simulink model "COSTEP"  (R2024b)
settings: Solver=FixedStepAuto  StartTime=0.0  StopTime=25  FixedStep=1/3600  RelTol=1e-3
model workspace (MAT data in the model file):
  AD = Simulink.Parameter
  AD.Value = [1; 1; 1; 23.3; 33.9; 32.8; 49.9; 50.5]
  AD.Complexity = 'real'
  AD.Dimensions = [8 1]
  AD.DataType = 'auto'
  AG = Simulink.Parameter
  AG.Value = [3.411e-06; 3.799e-07; 2.491e-07; 3.567e-07; 3.463e-07; 3.93e-07; 1.7e-07; 1.5e-07]
  AG.Complexity = 'real'
  AG.Dimensions = [8 1]
  AG.Description = 'Coefficient A to determine Enthalpy
    | MBtu/lb·°F'
  AG.DataType = 'auto'
  AH = Simulink.Parameter
  AH.Value = [1e-06; 1e-06; 1e-06; 9.6e-07; 5.73e-07; 6.52e-07; 5.15e-07; 4.71e-07]
  AH.Complexity = 'real'
  AH.Dimensions = [8 1]
  AH.Description = 'Coefficient C to determine Enthalpy
    | MBtu/lb·°F³'
  AH.DataType = 'auto'
  AV = Simulink.Parameter
  AV.Value = [1e-06; 1e-06; 1e-06; 8.67e-05; 0.00016; 0.00016; 0.000225; 0.000209]
  AV.Complexity = 'real'
  AV.Dimensions = [8 1]
  AV.DataType = 'auto'
  AVP = Simulink.Parameter
  AVP.Value = [0; 0; 0; 15.92; 16.35; 16.35; 16.43; 17.21]
  AVP.Complexity = 'real'
  AVP.Dimensions = [8 1]
  AVP.DataType = 'auto'
  BCHL = Simulink.Parameter
  BCHL.Value = [0; 0; 0; 2118895; 2331760; 2492349; 2279927; 2994129]
  BCHL.Complexity = 'real'
  BCHL.Dimensions = [8 1]
  BCHL.DataType = 'auto'
  BCHV = Simulink.Parameter
  BCHV.Value = [254278; 948838; 625079; 1822034; 1979455; 2321416; 1491254; 1822996]
  BCHV.Complexity = 'real'
  BCHV.Dimensions = [8 1]
  BCHV.DataType = 'auto'
  BD = Simulink.Parameter
  BD.Value = [0; 0; 0; -0.07; -0.0957; -0.0995; -0.0191; -0.0541]
  BD.Complexity = 'real'
  BD.Dimensions = [8 1]
  BD.DataType = 'auto'
  BDIST = Simulink.Parameter
  BDIST.Value = 0
  BDIST.Complexity = 'real'
  BDIST.Dimensions = [1 1]
  BDIST.DataType = 'auto'
  BG = Simulink.Parameter
  BG.Value = [7.18e-10; 1.08e-09; 1.36e-11; 8.51e-10; 8.96e-10; 1.02e-09; 0; 0]
  BG.Complexity = 'real'
  BG.Dimensions = [8 1]
  BG.Description = 'Coefficient B to determine Enthalpy
    | MBtu/lb·°F²'
  BG.DataType = 'auto'
  BH = Simulink.Parameter
  BH.Value = [0; 0; 0; 8.7e-09; 2.41e-09; 2.18e-09; 5.65e-10; 8.7e-10]
  BH.Complexity = 'real'
  BH.Dimensions = [8 1]
  BH.Description = 'Coefficient B to determine Enthalpy
    | MBtu/lb·°F²'
  BH.DataType = 'auto'
  BVP = Simulink.Parameter
  BVP.Value = [0; 0; 0; -1444; -2114; -2114; -2748; -3318]
  BVP.Complexity = 'real'
  BVP.Dimensions = [8 1]
  BVP.DataType = 'auto'
  CD = Simulink.Parameter
  CD.Value = [0; 0; 0; -0.0002; -0.000152; -0.000233; -0.000425; -0.00015]
  CD.Complexity = 'real'
  CD.Dimensions = [8 1]
  CD.DataType = 'auto'
  CDIST = Simulink.Parameter
  CDIST.Value = 0
  CDIST.Complexity = 'real'
  CDIST.Dimensions = [1 1]
  CDIST.DataType = 'auto'
  CG = Simulink.Parameter
  CG.Value = [6e-13; -3.98e-13; -3.93e-14; -3.12e-13; -3.27e-13; -3.12e-13; 0; 0]
  CG.Complexity = 'real'
  CG.Dimensions = [8 1]
  CG.DataType = 'auto'
  CH = Simulink.Parameter
  CH.Value = [0; 0; 0; 4.81e-11; 1.82e-11; 1.94e-11; 3.82e-12; 2.62e-12]
  CH.Complexity = 'real'
  CH.Dimensions = [8 1]
  CH.DataType = 'auto'
  CVP = Simulink.Parameter
  CVP.Value = [0; 0; 0; 259; 265.5; 265.5; 232.9; 249.6]
  CVP.Complexity = 'real'
  CVP.Dimensions = [8 1]
  CVP.DataType = 'auto'
  DDIST = Simulink.Parameter
  DDIST.Value = 0
  DDIST.Complexity = 'real'
  DDIST.Dimensions = [1 1]
  DDIST.DataType = 'auto'
  DIST_CONST = Simulink.Parameter
  DIST_CONST.Value = [0.2  0.5  0.03  0.485  0; 0.7  1  0.003  0.005  0; 0.25  0.5  10  45  0; 0.7  1  10  45  0; 0.15  0.25  10  35  0; 0.15  0.25  10  40  0; 1  2  0.25  1  0; 1  2  0.25  1  0; 0.4  0.5  0.25  0  0; 1.5  2  0  0  0; 2  3  0  0  0; 1.5  2  0  0  0; 0.15  0.25  10  45  0; 0.25  0.5  10  45  0; 0.15  0.25  5  100  0; 0.25  0.5  20  400  0; 0.25  0.5  20  400  0; 0.7  1  75  1500  0; 0.1  0.2  50  1000  0; 0.1  0.2  60  1200  0]
  DIST_CONST.Complexity = 'real'
  DIST_CONST.Dimensions = [20 5]
  DIST_CONST.Description = 'The random variation disturbances make use of disturbance parameters that are 
    | used to define the characteristics of the disturbances over time. 
    | These disturbance parameters are defined here as a matrix where each row corresponds 
    | to a different disturbance number, and where each column represents the different 
    | disturbance parameters, i.e. HSPAN, HZERO, SSPAN, SZERO, SPSPAN'
  DIST_CONST.DataType = 'auto'
  ISV = Simulink.Parameter
  ISV.Value = [10.40491 4.364 7.57006 0.423 24.15513 2.9426 154.3771 159.1866 2.80852 63.75581 26.74026 46.38532 ... (350 elements, 50x7)]
  ISV.Complexity = 'real'
  ISV.Dimensions = [50 7]
  ISV.Description = 'Initial state variable value for the different mode selections'
  ISV.DataType = 'auto'
  TLAST = Simulink.Parameter
  TLAST.Value = 0
  TLAST.Complexity = 'real'
  TLAST.Dimensions = [1 1]
  TLAST.DataType = 'auto'
  TNEXT = Simulink.Parameter
  TNEXT.Value = 0.1
  TNEXT.Complexity = 'real'
  TNEXT.Dimensions = [1 1]
  TNEXT.DataType = 'auto'
  XMW = Simulink.Parameter
  XMW.Value = [2; 25.4; 28; 32; 46; 48; 62; 76]
  XMW.Complexity = 'real'
  XMW.Dimensions = [8 1]
  XMW.Description = 'Molecular Weight of components lb/lb-mol'
  XMW.DataType = 'auto'
  XNS = Simulink.Parameter
  XNS.Value = [0.0012; 18; 22; 0.05; 0.2; 0.21; 0.3; 0.5; 0.01; 0.0017; 0.01; 1; 0.3; 0.125; 1; 0.3; 0.115; 0.01; 1.15; 0.2; 0.01; 0.01; 0.25; 0.1; 0.25; 0.1; 0.25; 0.025; 0.25; 0.1; 0.25; 0.1; 0.25; 0.025; 0.05; 0.05; 0.01; 0.01; 0.01; 0.5; 0.5]
  XNS.Complexity = 'real'
  XNS.Dimensions = [41 1]
  XNS.DataType = 'auto'
  XNS2 = Simulink.Parameter
  XNS2.Value = [0.25; 0.1; 0.25; 0.1; 0.25; 0.025; 0.25; 0.1; 0.25; 0.1; 0.25; 0.025; 0.05; 0.05]
  XNS2.Complexity = 'real'
  XNS2.Dimensions = [14 1]
  XNS2.DataType = 'auto'
  XNS3 = Simulink.Parameter
  XNS3.Value = [0.01; 0.01; 0.01; 0.5; 0.5]
  XNS3.Complexity = 'real'
  XNS3.Dimensions = [5 1]
  XNS3.DataType = 'auto'
  XNSADD = Simulink.Parameter
  XNSADD.Value = [0.01; 0.01; 0.01; 0.01; 0.01; 0.125; 0.01; 0.125; 0.01; 0.01; 0.25; 0.1; 0.25; 0.1; 0.25; 0.025; 0.25; 0.1; 0.25; 0.1; 0.25; 0.025; 0.25; 0.1; 0.25; 0.1; 0.25; 0.025; 0.25; 0.1; 0.25; 0.1; 0.25; 0.025]
  XNSADD.Complexity = 'real'
  XNSADD.Dimensions = [34 1]
  XNSADD.DataType = 'auto'
  XNSE = Simulink.Parameter
  XNSE.Value = [0.01; 0.3; 0.01; 0.3; 0.01; 0.3; 0.01; 0.3; 0.01; 0.2; 0.01; 0.2; 0.3; 0.3; 0.01; 0.3; 0.2; 0.01; 0.3; 0.01; 0.3; 0.2; 0.01; 0.3]
  XNSE.Complexity = 'real'
  XNSE.Dimensions = [24 1]
  XNSE.DataType = 'auto'
undefined symbols (not defined in the file or in its folder): magnitude, msgbox, SETPT, XMEAS, XMV
libraries: mylib x381, dspindex x31
(part 1 of 12)
settings Model: Creator=j3vos  LastModifiedBy=bligr
settings SolverCC: AlgebraicLoopSolver=TrustRegion
settings DataIOCC: ReturnWorkspaceOutputs=off
settings DebuggingCC: UnconnectedInputMsg=warning  UnconnectedOutputMsg=warning  UnconnectedLineMsg=warning  ArithmeticOperatorsInVariantConditions=warning
settings ModelReferenceCC: EnableRefExpFcnMdlSchedulingChecks=on
settings SFSimCC: SimUseLocalCustomCode=off  CustomCodeUndefinedFunction=UseInterfaceOnly
settings RTWCC: RTWUseLocalCustomCode=off  GPUComputeCapability=3.5

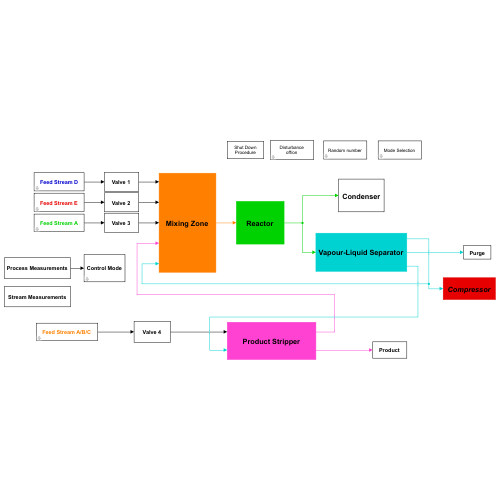
[thumbnail: Simulink's stored preview of the top-level diagram]
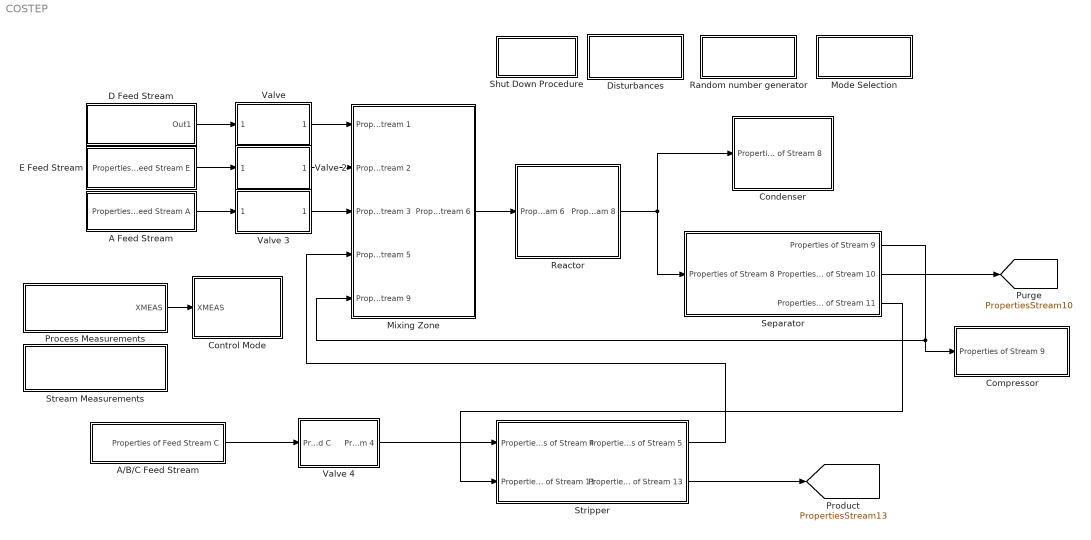
== system COSTEP ==
  A Feed Stream : Subsystem  mask{XST3_A=0.9999, XST3_B=0.0001, XST3_C=0, XST3_D=0, XST3_E=0, XST3_F=0, XST3_G=0, XST3_H=0, TST3=45, VRNG3=100}
      mask prompts: XST3_A "Fraction of A in Stream 3"; XST3_B "Fraction of B in Stream 3"; XST3_C "Fraction of C in Stream 3"; XST3_D "Fraction of D in Stream 3"; XST3_E "Fraction of E in Stream 3"; XST3_F "Fraction of F in Stream 3"; XST3_G "Fraction of G in Stream 3"; XST3_H "Fraction of H in Stream 3"; TST3 "Temperature of Stream 3"; VRNG3 "Maximum flow of Stream 3"
      mask DialogControl DescTextVar Prompt: Enter the Composition, Temperature and Mass Flow of Feed Stream A entering the plant
      mask DialogControl ParameterGroupVar Prompt: Properties of Feed Stream A
      mask Display: color('Green'),disp('{\bf\fontsize{12}Feed Stream A}', 'texmode','on');
  A/B/C Feed Stream : Subsystem  mask{XST4_A=0.485, XST4_B=0.005, XST4_C=0.51, XST4_D=0, XST4_E=0, XST4_F=0, XST4_G=0, XST4_H=0, TST4=45, VRNG4=1500}
      mask prompts: XST4_A "Fraction of A in Stream 4"; XST4_B "Fraction of B in Stream 4"; XST4_C "Fraction of C in Stream 4"; XST4_D "Fraction of D in Stream 4"; XST4_E "Fraction of E in Stream 4"; XST4_F "Fraction of F in Stream 4"; XST4_G "Fraction of G in Stream 4"; XST4_H "Fraction of H in Stream 4"; TST4 "Temperature of Stream 4"; VRNG4 "Maximum flow of Stream 4"
      mask DialogControl DescTextVar Prompt: Enter the Composition, Temperature and Mass Flow of Feed Stream C entering the plant
      mask DialogControl ParameterGroupVar Prompt: Properties of Feed Stream C
      mask Display: color('Orange'),disp('{\bf\fontsize{12}Feed Stream A/B/C}', 'texmode','on');
  Compressor : Subsystem
      mask Display: color('Black'),disp('{\bf\fontsize{16}Compressor}', 'texmode','on');
  Condenser : Subsystem
      mask Display: color('Black'),disp('{\bf\fontsize{16}Condenser}', 'texmode','on');
  Control Mode : Subsystem  mask{OPL=off, B=on, R=off, C=off, XMV1_0=63.053, XMV2_0=53.980, XMV3_0=24.644, XMV4_0=61.302, XMV5_0=22.210, XMV6_0=40.064, XMV7_0=38.100, XMV8_0=46.534, XMV9_0=47.446, XMV10_0=41.106, XMV11_0=18.114, XMV12_0=50.00000000}
      mask prompts: OPL "Open loop"; B "Braatz"; R "Ricker"; C "Custom"; XMV1_0 "Initial value of XMV(1) - D Feed flow valve"; XMV2_0 "Initial value of XMV(2) - E Feed flow valve"; XMV3_0 "Initial value of XMV(3) - A Feed flow valve"; XMV4_0 "Initial value of XMV(4) - A and C Feed flow valve"; XMV5_0 "Initial value of XMV(5) - Compressor recycle valve"; XMV6_0 "Initial value of XMV(6) - Purge valve"; XMV7_0 "Initial value of XMV(7) - Separator liquid flow valve"; XMV8_0 "Initial value of XMV(8) - Stripper liquid product flow valve"; XMV9_0 "Initial value of XMV(9) - Stripper steam valve"; XMV10_0 "Initial value of XMV(10) - Reactor cooling water flow valve"; XMV11_0 "Initial value of XMV(11) - Condenser cooling water flow valve"; XMV12_0 "Initial value of XMV(12) - Agitator speed"
      mask DialogControl DescGroupVar Prompt: Manipulated variables
      mask DialogControl DescTextVar Prompt: Control loops for manipulated variables. Open loop is the original TEP process without any control. Only one loop can be selected for a run. The base case values are the initial values of the manipulated variables
      mask DialogControl ParameterGroupVar Prompt: Control strategy
      mask DialogControl Container6 Prompt: Base case values
      mask Display: color('Black'),disp('{\bf\fontsize{12}Control Mode}', 'texmode','on');
  D Feed Stream : Subsystem  mask{XST1_A=0, XST1_B=0.0001, XST1_C=0, XST1_D=0.9999, XST1_E=0, XST1_F=0, XST1_G=0, XST1_H=0, TST1=45, VRNG1=400}
      mask prompts: XST1_A "Fraction of A in Stream 1"; XST1_B "Fraction of B in Stream 1"; XST1_C "Fraction of C in Stream 1"; XST1_D "Fraction of D in Stream 1"; XST1_E "Fraction of E in Stream 1"; XST1_F "Fraction of F in Stream 1"; XST1_G "Fraction of G in Stream 1"; XST1_H "Fraction of H in Stream 1"; TST1 "Temperature of Stream 1"; VRNG1 "Maximum flow of Stream 1"
      mask DialogControl DescTextVar Prompt: Enter the Composition, Temperature and Mass Flow of Feed Stream D entering the plant
      mask DialogControl ParameterGroupVar Prompt: Properties of Feed Stream D
      mask Display: color('Blue'),disp('{\bf\fontsize{12}Feed Stream D}', 'texmode','on');
  Disturbances : Subsystem  mask{DD=1, IDV1=off, IDV2=off, IDV3=off, IDV4=off, IDV5=off, IDV6=off, IDV7=off, IDV8=off, IDV9=off, IDV10=off, IDV11=off, IDV12=off, IDV13=off, IDV14=off, IDV15=off, IDV16=off, IDV17=off, IDV18=off, IDV19=off, IDV20=off, IDV21=off, IDV22=off, IDV23=off, IDV24=off, IDV25=off, IDV26=off, IDV27=off, IDV28=off}
      mask prompts: DD "Simulation time when disturbances should be introduced (in hours)"; IDV1 "IDV(1) - A/C feed ratio"; IDV2 "IDV(2) - B composition"; IDV3 "IDV(3) - D feed temperature"; IDV4 "IDV(4) - Reactor cooling water inlet temperature"; IDV5 "IDV(5) - Condenser cooling water inlet temperature"; IDV6 "IDV(6) - A feed loss"; IDV7 "IDV(7) - C header pressure loss (reduced availability)"; IDV8 "IDV(8) - A, B, C feed composition"; IDV9 "IDV(9) - D feed temperature"; IDV10 "IDV(10) - C feed temperature"; IDV11 "IDV(11) - Reactor cooling water inlet temperature"; IDV12 "IDV(12) - Condenser cooling water inlet temperature"; IDV13 "IDV(13) - Reaction kinetics"; IDV14 "IDV(14) - Reactor cooling water valve"; IDV15 "IDV(15) - Condenser cooling water valve"; IDV16 "IDV(16) - Unknown"; IDV17 "IDV(17) - Unknown"; IDV18 "IDV(18) - Unknown"; IDV19 "IDV(19) - Unknown"; IDV20 "IDV(20) - Unknown"; IDV21 "IDV(21) - A feed temperature"; IDV22 "IDV(22) - E feed temperature"; IDV23 "IDV(23) - A feed pressure"; IDV24 "IDV(24) - D feed pressure"; IDV25 "IDV(25) - E feed pressure"; IDV26 "IDV(26) - A, B, C feed pressure"; IDV27 "IDV(27) - Reactor cooling water supply pressure"; IDV28 "IDV(28) - Condensor cooling water supply pressure"
      mask DialogControl DescTextVar Prompt: Indicate if any disturbances are present (more than one can be ticked at a time)
      mask DialogControl ParameterGroupVar Prompt: Disturbances
      mask Display: color('Black'),disp('Disturbance\noff/on')
  E Feed Stream : Subsystem  mask{XST2_A=0, XST2_B=0, XST2_C=0, XST2_D=0, XST2_E=0.9999, XST2_F=0.0001, XST2_G=0, XST2_H=0, TST2=45, VRNG2=400}
      mask prompts: XST2_A "Fraction of A in Stream 2"; XST2_B "Fraction of B in Stream 2"; XST2_C "Fraction of C in Stream 2"; XST2_D "Fraction of D in Stream 2"; XST2_E "Fraction of E in Stream 2"; XST2_F "Fraction of F in Stream 2"; XST2_G "Fraction of G in Stream 2"; XST2_H "Fraction of H in Stream 2"; TST2 "Temperature of Stream 2"; VRNG2 "Maximum flow of Stream 2"
      mask DialogControl DescTextVar Prompt: Enter the Composition, Temperature and Mass Flow of Feed Stream E entering the plant
      mask DialogControl ParameterGroupVar Prompt: Properties of Feed Stream E
      mask Display: color('Red'),disp('{\bf\fontsize{12}Feed Stream E}', 'texmode','on');
  Mixing Zone : Subsystem
      mask Display: color('Black'),disp('{\bf\fontsize{16}Mixing Zone}', 'texmode','on');
  Mode Selection : Subsystem  mask{M=Mode - Original}
      mask prompts: M "Mode selection"
      mask DialogControl DescTextVar Prompt: Enter the mode for simulation run
      mask Display: disp('Mode Selection')
  Process Measurements : Subsystem
      mask Display: color('Black'),disp('{\bf\fontsize{12}Process Measurements}', 'texmode','on');
  Random number generator : Subsystem  mask{G=4243534565}
      mask prompts: G "Random number seed"
      mask DialogControl DescTextVar Prompt: Enter a random number so that every runs results will differ
      mask DialogControl ParameterGroupVar Prompt: Random Number Generator
      mask Display: disp('Random number')
  Reactor : Subsystem
      mask Display: color('Black'),disp('{\bf\fontsize{16}Reactor}', 'texmode','on');
  Separator : Subsystem
      mask Display: color('Black'),disp('{\bf\fontsize{16}Vapour-Liquid Separator}', 'texmode','on');
  Shut Down Procedure : Subsystem
      mask Display: color('black'),disp('Shut Down\nProcedure')
  Stream Measurements : Subsystem
      mask Display: color('Black'),disp('{\bf\fontsize{12}Stream Measurements}', 'texmode','on');
  Stripper : Subsystem
      mask Display: color('Black'),disp('{\bf\fontsize{16}Product Stripper}', 'texmode','on');
  Valve : Subsystem
      mask Display: color('Black'),disp('{\bf\fontsize{12}Valve 1}', 'texmode','on');
  Valve 2 : Subsystem
      mask Display: color('Black'),disp('{\bf\fontsize{12}Valve 2}', 'texmode','on');
  Valve 3 : Subsystem
      mask Display: color('Black'),disp('{\bf\fontsize{12}Valve 3}', 'texmode','on');
  Valve 4 : Subsystem
      mask Display: color('Black'),disp('{\bf\fontsize{12}Valve 4}', 'texmode','on');
  tag scope: PropertiesStream10=global, PropertiesStream13=global
  wires:
  Valve/1(Properties of Stream 1) -> Mixing Zone/1(Properties of Stream 1)
  E Feed Stream/1("Properties of Feed Stream E ") -> Valve 2/1(Properties of Feed E)
  Valve 2/1(Properties of Stream 2) -> Mixing Zone/2(Properties of Stream 2)
  A Feed Stream/1("Properties of Feed Stream A ") -> Valve 3/1(Properties of Feed A)
  Valve 3/1(Properties of Stream 3) -> Mixing Zone/3(Properties of Stream 3)
  Stripper/1(Properties of Stream 5) -> Mixing Zone/4(Properties of Stream 5)
  Mixing Zone/1(Properties of Stream 6) -> Reactor/1(Properties of Stream 6)
  A/B/C Feed Stream/1("Properties of Feed Stream C ") -> Valve 4/1(Properties of Feed C)
  Valve 4/1(Properties of Stream 4) -> Stripper/1(Properties of Stream 4)
  Separator/3(Properties of Stream 11) -> Stripper/2(Properties of Stream 11)
  Reactor/1(Properties of Stream 8) -> Separator/1(Properties of Stream 8), Condenser/1(Properties of Stream 8)
  Separator/1(Properties of Stream 9) -> Compressor/1(Properties of Stream 9), Mixing Zone/5(Properties of Stream 9)
  D Feed Stream/1(Out1) -> Valve/1(Properties of Feed D)
  Process Measurements/1(XMEAS) -> Control Mode/1(XMEAS)
  Stripper/2(Properties of Stream 13) -> [PropertiesStream13]
  Separator/2(Properties of Stream 10) -> [PropertiesStream10]

== system COSTEP/A Feed Stream ==
  Bus Creator : BusCreator  Inputs=4
  HST(3) Molar Enthalpy of Stream 3 MBtu/lb-mol : Subsystem
  TST(3) Temperature of Stream 3 °C : Subsystem
  VRNG(3) Max flow of Stream 3 through valve lb-mol/h : Subsystem
  XST(I,3) Composition of Stream 3 : Constant  Value=[XST3_A;XST3_B;XST3_C;XST3_D;XST3_E;XST3_F;XST3_G;XST3_H]
  "Properties of Feed Stream A " : Outport  VectorParamsAs1DForOutWhenUnconnected=off
  wires:
  XST(I,3) Composition of Stream 3/1 -> HST(3) Molar Enthalpy of Stream 3 MBtu/lb-mol/2(XST(I,3)), Bus Creator/1  "XST(I;3)"
  TST(3) Temperature of Stream 3 °C/1(TST(3)) -> HST(3) Molar Enthalpy of Stream 3 MBtu/lb-mol/1(TST(3)), Bus Creator/2  "TST(3)"
  VRNG(3) Max flow of Stream 3 through valve lb-mol/h/1(VRNG(3)) -> Bus Creator/3  "VRNG(3)"
  HST(3) Molar Enthalpy of Stream 3 MBtu/lb-mol/1(HST(3)) -> Bus Creator/4  "HST(3)"
  Bus Creator/1 -> "Properties of Feed Stream A "/1

== system COSTEP/A//B//C Feed Stream ==
  note: TST(4)
      | Temperature of Stream 4
      | °C
  Bus Creator : BusCreator  Inputs=4
  Bus Selector : BusSelector  OutputSignals=signal1.TESUB8(1),signal1.TESUB8(2)
  Bus Selector1 : BusSelector  OutputSignals=IDV(1),IDV(2)
  Bus Selector2 : BusSelector  OutputSignals=signal1.TESUB8(4)
  Gain : Gain
  HST(4) Molar Enthalpy of Stream 4 MBtu/lb-mol : Subsystem
  VRNG(4) Max flow of Stream 4 through valve lb-mol/h : Subsystem
  "XST(I;4) Composition of Stream 4 " : Subsystem
  "Properties of Feed Stream C " : Outport  VectorParamsAs1DForOutWhenUnconnected=off
  wires:
  "XST(I;4) Composition of Stream 4 "/1(XST(I;4)) -> HST(4) Molar Enthalpy of Stream 4 MBtu/lb-mol/2(XST(I,4)), Bus Creator/1  "XST(I;4)"
  Bus Selector2/1 -> Gain/1, HST(4) Molar Enthalpy of Stream 4 MBtu/lb-mol/1(TST(4))  "<TESUB8(4)>"
  VRNG(4) Max flow of Stream 4 through valve lb-mol/h/1(VRNG(4)) -> Bus Creator/3  "VRNG(4)"
  Bus Creator/1 -> "Properties of Feed Stream C "/1
  HST(4) Molar Enthalpy of Stream 4 MBtu/lb-mol/1(HST(4)) -> Bus Creator/4  "HST(4)"
  Bus Selector/2 -> "XST(I;4) Composition of Stream 4 "/2(TESUB8(2))  "<TESUB8(2)>"
  [TESUB8] -> Bus Selector2/1, Bus Selector/1
  Bus Selector/1 -> "XST(I;4) Composition of Stream 4 "/1(TESUB8(1))  "<TESUB8(1)>"
  [IDV] -> Bus Selector1/1
  Bus Selector1/1 -> "XST(I;4) Composition of Stream 4 "/3(IDV(1))  "<IDV(1)>"
  Bus Selector1/2 -> "XST(I;4) Composition of Stream 4 "/4(IDV(2))  "<IDV(2)>"
  Gain/1 -> Bus Creator/2  "TST(4)"

== system COSTEP/Compressor ==
  Properties of Stream 9 : Inport
  "  " : Subsystem
  Bus Selector : BusSelector  OutputSignals=XMWS(9)
  CPDH Compressor work MBtu/h : Subsystem
  CPFLMX : Constant  Value=280275
  Subsystem : Subsystem
  Subsystem1 : Subsystem
  TKS Temperature of Separator K : Sum
  To Convert °C to K : Constant  Value=273.15
  tag scope: CPDH=global, FLMS=global
  wires:
  Subsystem1/1(FLCOEF) -> "  "/3(FLCOEF)
  Subsystem/1(PR) -> "  "/1(PR)
  CPFLMX/1 -> "  "/2(CPFLMX), Subsystem1/1(CPFLMX)
  CPDH Compressor work MBtu/h/1(CPDH) -> [CPDH]
  "  "/1(FLMS) -> [FLMS], CPDH Compressor work MBtu/h/1(FLMS)
  TKS Temperature of Separator K/1 -> CPDH Compressor work MBtu/h/2(TKS)
  [TCS] -> TKS Temperature of Separator K/1
  To Convert °C to K/1 -> TKS Temperature of Separator K/2
  Properties of Stream 9/1 -> Bus Selector/1
  Bus Selector/1 -> CPDH Compressor work MBtu/h/3("XMWS(9) ")  "<XMWS(9)>"

== system COSTEP/Condenser ==
  Properties of Stream 8 : Inport
  Cooling water outlet temperature : Subsystem
  FWS Flow of cooling water to Condenser Gallons per minute : Subsystem
  Position of Valve 11 % : Subsystem
  Subsystem : Subsystem
  VRNG(11) Max flow of water through valve Gallons per minute : Subsystem
  tag scope: FWS=global, QUS=global
  wires:
  VRNG(11) Max flow of water through valve Gallons per minute/1(VRNG(11)) -> FWS Flow of cooling water to Condenser Gallons per minute/2(VRNG(11))
  FWS Flow of cooling water to Condenser Gallons per minute/1(FWS) -> [FWS], Cooling water outlet temperature/1(FWS)
  Position of Valve 11 %/1("YY(49) ") -> FWS Flow of cooling water to Condenser Gallons per minute/1(VPOS(11))
  Subsystem/1("QUS ") -> Cooling water outlet temperature/2(QUS), [QUS]
  Properties of Stream 8/1 -> Subsystem/1(Properties of Stream 8)
  Cooling water outlet temperature/1("YY(38) ") -> Subsystem/2(TWS)

== system COSTEP/Control Mode ==
  XMEAS : Inport
  Braatz : Subsystem
  Constant : Constant  Value=OPL
  Constant1 : Constant  Value=B
  Constant2 : Constant  Value=R
  Constant3 : Constant  Value=C
  Custom Controller : Subsystem
  Custom Controller1 : Subsystem
  If : If  NumInputs=4  IfExpression=u1 == 1  ElseIfExpressions=u2 == 1, u3 == 1, u4 == 1  ShowElse=off
  If Action Subsystem : Subsystem  TreatAsAtomicUnit=on
  If Action Subsystem1 : Subsystem  TreatAsAtomicUnit=on
  If Action Subsystem2 : Subsystem  TreatAsAtomicUnit=on
  If Action Subsystem3 : Subsystem  TreatAsAtomicUnit=on
  Merge : Merge  Inputs=4
  Open loop : Subsystem
  Subsystem : Subsystem
      mask Display: color('Black'),disp('Multi loop\nselection')
  To Workspace2 : ToWorkspace  VariableName=XMV  SampleTime=-1
  tag scope: XMV=global
  wires:
  Constant/1 -> Subsystem/1(OPL), If/1
  Constant1/1 -> Subsystem/2(B), If/2
  Constant2/1 -> Subsystem/3(R), If/3
  Merge/1 -> [XMV], To Workspace2/1
  If/1 -> If Action Subsystem/Action
  Open loop/1(XMV) -> If Action Subsystem/1(In1)
  If Action Subsystem1/1(Out1) -> Merge/2
  If/2 -> If Action Subsystem1/Action
  If/3 -> If Action Subsystem2/Action
  If Action Subsystem/1(Out1) -> Merge/1
  If Action Subsystem2/1(Out1) -> Merge/3
  Braatz/1(XMV) -> If Action Subsystem1/1(In1)
  Custom Controller1/1(XMV) -> If Action Subsystem2/1(In1)
  XMEAS/1 -> Braatz/1(XMEAS)
  If/4 -> If Action Subsystem3/Action
  Constant3/1 -> Subsystem/4(C), If/4
  Custom Controller/1(XMV) -> If Action Subsystem3/1(XMV)
  If Action Subsystem3/1(Out1) -> Merge/4

== system COSTEP/D Feed Stream ==
  Bus Creator : BusCreator  Inputs=4
  HST(1) Molar Enthalpy of Stream 1 MBtu/lb-mol : Subsystem
  TST(1) Temperature of Stream 1 °C : Subsystem
  VRNG(1) Max flow of Stream 1 through valve lb-mol/h : Subsystem
  XST(I,1) Composition of Stream 1 : Constant  Value=[XST1_A;XST1_B;XST1_C;XST1_D;XST1_E;XST1_F;XST1_G;XST1_H]
  Out1 : Outport  VectorParamsAs1DForOutWhenUnconnected=off
  wires:
  XST(I,1) Composition of Stream 1/1 -> HST(1) Molar Enthalpy of Stream 1 MBtu/lb-mol/2(XST(I,1)), Bus Creator/1  "XST(I;1)"
  VRNG(1) Max flow of Stream 1 through valve lb-mol/h/1(VRNG(1)) -> Bus Creator/3  "VRNG(1)"
  HST(1) Molar Enthalpy of Stream 1 MBtu/lb-mol/1(HST(1)) -> Bus Creator/4  "HST(1)"
  TST(1) Temperature of Stream 1 °C/1(TST(1)) -> Bus Creator/2, HST(1) Molar Enthalpy of Stream 1 MBtu/lb-mol/1(TST(1))
  Bus Creator/1 -> Out1/1

== system COSTEP/Disturbances ==
  Constant : Constant  Value=DD
  Delay : Delay  DelayLengthSource=Input port  DelayLength=1  DelayLengthUpperLimit=DD*3600  InitialCondition=0
      settings: InputPortMap=u0,p1
  Gain : Gain  Gain=3600
  IDV bus signal : Subsystem
  IDV from check box : Subsystem
  MATLAB Function : MATLAB Function  TreatAsAtomicUnit=on
  tag scope: IDV=global
  wires:
  Constant/1 -> Gain/1
  Gain/1 -> Delay/2
  Delay/1 -> [IDV]
  IDV from check box/1(Out1) -> MATLAB Function/1(IDV)
  MATLAB Function/1(IDV_out) -> IDV bus signal/1(IDV)
  IDV bus signal/1(Out1) -> Delay/1

== system COSTEP/E Feed Stream ==
  Bus Creator : BusCreator  Inputs=4
  HST(2) Molar Enthalpy of Stream 2 MBtu/lb-mol : Subsystem
  TST(2) Temperature of Stream 2 °C : Subsystem
  VRNG(2) Max flow of Stream 2 through valve lb-mol/h : Subsystem
  XST(I,2) Composition of Stream 2 : Constant  Value=[XST2_A;XST2_B;XST2_C;XST2_D;XST2_E;XST2_F;XST2_G;XST2_H]
  "Properties of Feed Stream E " : Outport  VectorParamsAs1DForOutWhenUnconnected=off
  wires:
  XST(I,2) Composition of Stream 2/1 -> HST(2) Molar Enthalpy of Stream 2 MBtu/lb-mol/2(XST(I,2)), Bus Creator/1  "XST(I;2)"
  TST(2) Temperature of Stream 2 °C/1(TST(2)) -> HST(2) Molar Enthalpy of Stream 2 MBtu/lb-mol/1(TST(2)), Bus Creator/2  "TST(2)"
  VRNG(2) Max flow of Stream 2 through valve lb-mol/h/1(VRNG(2)) -> Bus Creator/3  "VRNG(2)"
  Bus Creator/1 -> "Properties of Feed Stream E "/1
  HST(2) Molar Enthalpy of Stream 2 MBtu/lb-mol/1(HST(2)) -> Bus Creator/4  "HST(2)"

== system COSTEP/Mixing Zone ==
  Properties of Stream 1 : Inport
  Properties of Stream 2 : Inport  Port=2
  Properties of Stream 3 : Inport  Port=3
  Properties of Stream 5 : Inport  Port=4
  Properties of Stream 9 : Inport  Port=5
  Bus Creator : BusCreator  Inputs=2
  ETV Internal energy of Mixing zone Btu : Gain
  Holdup of Components in Mixing Zone : Subsystem
  Internal energy of mixing zone : Subsystem
  PTV Total pressure of Mixing zone mmHg : Subsystem
  Stream 6 : Subsystem
  "TCV Initial Temperature in Mixing zone °C " : Subsystem
  Properties of Stream 6 : Outport  VectorParamsAs1DForOutWhenUnconnected=off
  tag scope: PTV=global, PropertiesStream6=global
  wires:
  "TCV Initial Temperature in Mixing zone °C "/1(TCV) -> PTV Total pressure of Mixing zone mmHg/2(TCV), Stream 6/2(TST(6))
  Internal energy of mixing zone/1("YY(36) ") -> ETV Internal energy of Mixing zone Btu/1
  Properties of Stream 1/1 -> Holdup of Components in Mixing Zone/1(Properties of Stream 1), Internal energy of mixing zone/1(Properties of Stream 1)
  Properties of Stream 2/1 -> Internal energy of mixing zone/2(Properties of Stream 2), Holdup of Components in Mixing Zone/2(Properties of Stream 2)
  Properties of Stream 3/1 -> Internal energy of mixing zone/3(Properties of Stream 3), Holdup of Components in Mixing Zone/3(Properties of Stream 3)
  Stream 6/1(Properties of Stream 6) -> Bus Creator/1, Properties of Stream 6/1
  Properties of Stream 5/1 -> Internal energy of mixing zone/4(Properties of Stream 5), Holdup of Components in Mixing Zone/4(Properties of Stream 5)
  Properties of Stream 9/1 -> Internal energy of mixing zone/5(Properties of Stream 9), Holdup of Components in Mixing Zone/5(Properties of Stream 9)
  Holdup of Components in Mixing Zone/1(XVV) -> Stream 6/1(XST(I,6)), "TCV Initial Temperature in Mixing zone °C "/3(XVV)
  Holdup of Components in Mixing Zone/2(UTVV) -> PTV Total pressure of Mixing zone mmHg/1(UTVV), "TCV Initial Temperature in Mixing zone °C "/1(UTVV)
  PTV Total pressure of Mixing zone mmHg/1(PTV) -> Bus Creator/2, [PTV]  "PTV"
  Bus Creator/1 -> [PropertiesStream6]
  ETV Internal energy of Mixing zone Btu/1 -> "TCV Initial Temperature in Mixing zone °C "/2(ETV)

== system COSTEP/Mode Selection ==
  Constant : Constant  Value=M
  MATLAB Function : MATLAB Function  TreatAsAtomicUnit=on
  tag scope: M=global
  wires:
  Constant/1 -> MATLAB Function/1(M)
  MATLAB Function/1(M_out) -> [M]

== system COSTEP/Process Measurements ==
  Bus Creator1 : BusCreator  Inputs=10
  Compressor Work : Subsystem
  Condenser Cooling Outlet Water Temperature : Subsystem
  Feed Streams : Subsystem
  Product analysis : Subsystem
  Purge gas analysis : Subsystem
  Reactor Cooling Outlet Water Temperature : Subsystem
  Reactor feed analysis : Subsystem
  Subsystem3 : Subsystem
  Subsystem4 : Subsystem
  Subsystem5 : Subsystem
  To Workspace1 : ToWorkspace  VariableName=XMEAS  SampleTime=-1
  XMEAS : Outport  VectorParamsAs1DForOutWhenUnconnected=off
  tag scope: XMEAS=global
  wires:
  Bus Creator1/1 -> To Workspace1/1, [XMEAS], XMEAS/1
  Feed Streams/1(XMEASF) -> Bus Creator1/1
  Subsystem3/1(Reactor) -> Bus Creator1/2
  Subsystem4/1(Separator) -> Bus Creator1/3
  Subsystem5/1(Stripper) -> Bus Creator1/4
  Product analysis/1(XMEAS) -> Bus Creator1/10
  Purge gas analysis/1(XMEASP) -> Bus Creator1/9
  Reactor feed analysis/1(XMEASR) -> Bus Creator1/8
  Compressor Work/1("XMEAS(20) ") -> Bus Creator1/5
  Reactor Cooling Outlet Water Temperature/1(XMEAS(21)) -> Bus Creator1/6
  Condenser Cooling Outlet Water Temperature/1(XMEAS(22)) -> Bus Creator1/7

== system COSTEP/Random number generator ==
  Additional Stream Measurements : Delay  DelayLength=1  InitialConditionSource=Input port  InitialCondition=0
      settings: InputPortMap=u0,p4
  Bus Creator : BusCreator  Inputs=3
  Constant : Constant  Value=G
  "Disturbances 17, 18, 20 IDVWLK=10-12" : Subsystem
  "Disturbances 21, 22, 23, 24, 25, 26, 27, 28 IDVWLK=13-20" : Subsystem
  "Disturbances 8, 9, 10, 11, 12, 13, 16 IDVWLK=1-9" : Subsystem
  MATLAB Function : MATLAB Function  TreatAsAtomicUnit=on
  Original G : Delay  DelayLength=1  InitialConditionSource=Input port  InitialCondition=0
      settings: InputPortMap=u0,p4
  Process Disturbances : Delay  DelayLength=1  InitialConditionSource=Input port  InitialCondition=0
      settings: InputPortMap=u0,p4
  Process Measurements XMEAS(I) I=1-22 : Subsystem
  Process Measurements XMEAS(I) I=23-36 : Subsystem
  Process Measurements XMEAS(I) I=37-41 : Subsystem
  Stream Measurements SMEAS Gas analysis1 : Subsystem
  Stream Measurements SMEAS Product analysis1 : Subsystem
  Stream Measurements SMEAS1 : Subsystem
  tag scope: TESUB8=global
  wires:
  "Disturbances 17, 18, 20 IDVWLK=10-12"/1(G2) -> Process Measurements XMEAS(I) I=1-22/1(G2)
  Process Measurements XMEAS(I) I=37-41/1(G5) -> Original G/1
  Process Measurements XMEAS(I) I=1-22/1(G3) -> Process Measurements XMEAS(I) I=23-36/1(G3)
  Process Measurements XMEAS(I) I=23-36/1(G4) -> Process Measurements XMEAS(I) I=37-41/1(G4)
  "Disturbances 8, 9, 10, 11, 12, 13, 16 IDVWLK=1-9"/1(G1) -> "Disturbances 17, 18, 20 IDVWLK=10-12"/1(G1)
  Original G/1 -> "Disturbances 8, 9, 10, 11, 12, 13, 16 IDVWLK=1-9"/1(G)
  Bus Creator/1 -> [TESUB8]
  "Disturbances 8, 9, 10, 11, 12, 13, 16 IDVWLK=1-9"/2(Out1) -> Bus Creator/1
  "Disturbances 17, 18, 20 IDVWLK=10-12"/2(Out1) -> Bus Creator/2
  "Disturbances 21, 22, 23, 24, 25, 26, 27, 28 IDVWLK=13-20"/1(G1) -> Process Disturbances/1
  Process Disturbances/1 -> "Disturbances 21, 22, 23, 24, 25, 26, 27, 28 IDVWLK=13-20"/1(G)
  Constant/1 -> MATLAB Function/1(G)
  Stream Measurements SMEAS Product analysis1/1(GE4) -> Additional Stream Measurements/1
  Stream Measurements SMEAS1/1(G2E) -> Stream Measurements SMEAS Gas analysis1/1(GE2)
  Stream Measurements SMEAS Gas analysis1/1(GE3) -> Stream Measurements SMEAS Product analysis1/1(GE3)
  Additional Stream Measurements/1 -> Stream Measurements SMEAS1/1(G1E)
  MATLAB Function/1(G_out) -> Additional Stream Measurements/2, Process Disturbances/2, Original G/2
  "Disturbances 21, 22, 23, 24, 25, 26, 27, 28 IDVWLK=13-20"/2(Out1) -> Bus Creator/3

== system COSTEP/Reactor ==
  Properties of Stream 6 : Inport
  Bus Creator : BusCreator  Inputs=2
  Holdup of Components in Reactor : Subsystem
  Internal energy of reactor : Subsystem
  Pressure of Reactor : Subsystem
  Reaction Rates : Subsystem
  Reactor Heat exchanger : Subsystem
  Stream 8 : Subsystem
  "TCR Initial Temperature in Reactor °C " : Subsystem
  Total Vapour Component Holdup in Reactor : Subsystem
  Vapour Component Fraction in Reactor : Subsystem
  Volume of Reactor : Subsystem
  Properties of Stream 8 : Outport  VectorParamsAs1DForOutWhenUnconnected=off
  tag scope: PTR=global, PropertiesStream8=global, TCR=global, VLR=global
  wires:
  Holdup of Components in Reactor/1(UTLR) -> Volume of Reactor/2(UTLR), "TCR Initial Temperature in Reactor °C "/1(UTLR)
  Internal energy of reactor/1("YY(9) ") -> "TCR Initial Temperature in Reactor °C "/2(ETR)  "ETR Internal energy of reactor MBtu"
  Stream 8/1(Properties of Stream 8) -> Bus Creator/1, Properties of Stream 8/1
  Reactor Heat exchanger/1(QUR) -> Internal energy of reactor/2(QUR)
  Properties of Stream 6/1 -> Holdup of Components in Reactor/2(Properties of Stream 6), Internal energy of reactor/3(Properties of Stream 6)
  Reaction Rates/1("RH ") -> Internal energy of reactor/1(RH)
  Reaction Rates/2(CRXR) -> Holdup of Components in Reactor/1(CRXR)
  Holdup of Components in Reactor/2(XLR) -> Pressure of Reactor/1(XLR), "TCR Initial Temperature in Reactor °C "/3(XLR), Volume of Reactor/1(XLR)
  Holdup of Components in Reactor/3(UCVR) -> Pressure of Reactor/3(UCVR)
  Pressure of Reactor/2(PPR) -> Reaction Rates/2(PPR), Vapour Component Fraction in Reactor/1(PPR)
  Pressure of Reactor/1(PTR) -> Bus Creator/2, [PTR]  "PTR"
  "TCR Initial Temperature in Reactor °C "/1(TCR) -> Stream 8/1(TST(8)), [TCR]
  Volume of Reactor/1(VVR) -> Reaction Rates/1(VVR), Total Vapour Component Holdup in Reactor/1(VVR), Pressure of Reactor/2(VVR)
  Vapour Component Fraction in Reactor/1(XVR) -> Total Vapour Component Holdup in Reactor/2(XVR), Stream 8/2(XTS(I,8))
  Volume of Reactor/2(VLR) -> [VLR]
  Bus Creator/1 -> [PropertiesStream8]

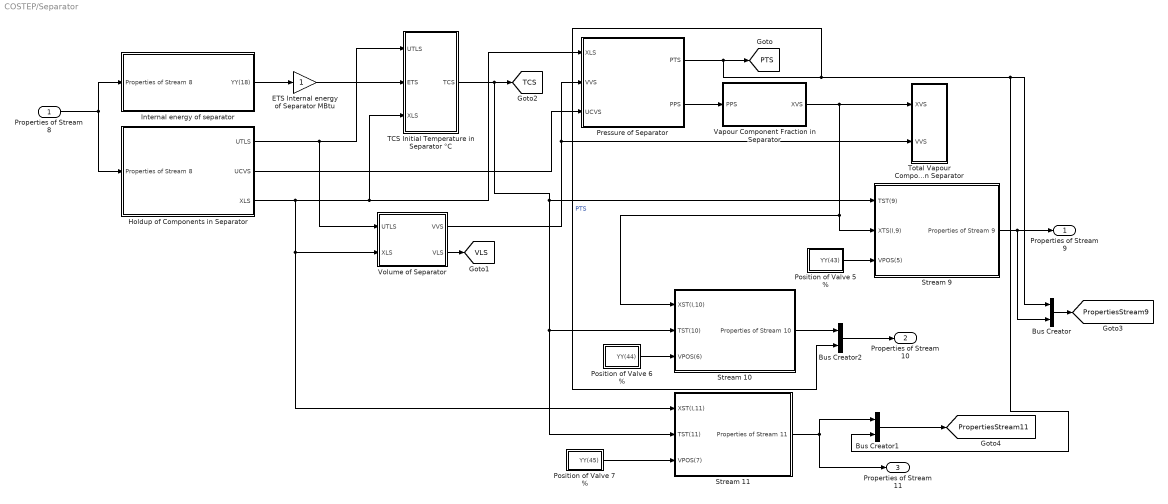
== system COSTEP/Separator ==
  Properties of Stream 8 : Inport
  Bus Creator : BusCreator  Inputs=2
  Bus Creator1 : BusCreator  Inputs=2
  Bus Creator2 : BusCreator  Inputs=2
  ETS Internal energy of Separator MBtu : Gain
  Holdup of Components in Separator : Subsystem
  Internal energy of separator : Subsystem
  Position of Valve 5 % : Subsystem
  Position of Valve 6 % : Subsystem
  Position of Valve 7 % : Subsystem
  Pressure of Separator : Subsystem
  Stream 10 : Subsystem
  Stream 11 : Subsystem
  Stream 9 : Subsystem
  "TCS Initial Temperature in Separator °C " : Subsystem
  Total Vapour Component Holdup in Separator : Subsystem
  Vapour Component Fraction in Separator : Subsystem
  Volume of Separator : Subsystem
  Properties of Stream 9 : Outport  VectorParamsAs1DForOutWhenUnconnected=off
  Properties of Stream 10 : Outport  Port=2  VectorParamsAs1DForOutWhenUnconnected=off
  Properties of Stream 11 : Outport  Port=3  VectorParamsAs1DForOutWhenUnconnected=off
  tag scope: PTS=global, PropertiesStream11=global, PropertiesStream9=global, TCS=global, VLS=global
  wires:
  Internal energy of separator/1("YY(18) ") -> ETS Internal energy of Separator MBtu/1
  Stream 9/1(Properties of Stream 9) -> Bus Creator/2, Properties of Stream 9/1
  Stream 11/1(Properties of Stream 11) -> Bus Creator1/1, Properties of Stream 11/1
  Holdup of Components in Separator/1(UTLS) -> Volume of Separator/1(UTLS), "TCS Initial Temperature in Separator °C "/1(UTLS)
  Holdup of Components in Separator/3(XLS) -> "TCS Initial Temperature in Separator °C "/3(XLS), Pressure of Separator/1(XLS), Stream 11/1(XST(I,11)), Volume of Separator/2(XLS)
  Volume of Separator/1(VVS) -> Pressure of Separator/2(VVS), Total Vapour Component Holdup in Separator/2(VVS)
  Volume of Separator/2(VLS) -> [VLS]
  Pressure of Separator/1(PTS) -> Bus Creator2/2, Bus Creator1/2, Bus Creator/1, [PTS]  "PTS"
  Holdup of Components in Separator/2(UCVS) -> Pressure of Separator/3(UCVS)
  Vapour Component Fraction in Separator/1(XVS) -> Stream 10/1(XST(I,10)), Stream 9/2(XTS(I,9)), Total Vapour Component Holdup in Separator/1(XVS)
  Pressure of Separator/2(PPS) -> Vapour Component Fraction in Separator/1(PPS)
  Properties of Stream 8/1 -> Internal energy of separator/1(Properties of Stream 8), Holdup of Components in Separator/1(Properties of Stream 8)
  Position of Valve 5 %/1("YY(43) ") -> Stream 9/3(VPOS(5))
  Position of Valve 6 %/1("YY(44) ") -> Stream 10/3(VPOS(6))
  Position of Valve 7 %/1("YY(45) ") -> Stream 11/3(VPOS(7))
  ETS Internal energy of Separator MBtu/1 -> "TCS Initial Temperature in Separator °C "/2(ETS)
  "TCS Initial Temperature in Separator °C "/1(TCS) -> [TCS], Stream 11/2(TST(11)), Stream 10/2(TST(10)), Stream 9/1(TST(9))
  Bus Creator/1 -> [PropertiesStream9]
  Bus Creator1/1 -> [PropertiesStream11]
  Stream 10/1(Properties of Stream 10) -> Bus Creator2/1
  Bus Creator2/1 -> Properties of Stream 10/1

== system COSTEP/Shut Down Procedure ==
  Add : Sum  Inputs=8  OutDataTypeStr=double  AccumDataTypeStr=double
  Reactor Level to High : Subsystem
  Reactor Level to Low : Subsystem
  Reactor Presssure to High : Subsystem
  Reactor Temperature to High : Subsystem
  Separator Level to High : Subsystem
  Separator Level to Low : Subsystem
  Stripper Level to High : Subsystem
  Stripper Level to Low : Subsystem
  tag scope: ISD=global
  wires:
  [VLR] -> Reactor Level to Low/1(VLR), Reactor Level to High/1(VLR)
  [VLS] -> Separator Level to Low/1(VLS), Separator Level to High/1(VLS)
  [VLC] -> Stripper Level to Low/1(VLC), Stripper Level to High/1(VLC)
  Reactor Presssure to High/1(ISD) -> Add/1
  Reactor Temperature to High/1(ISD) -> Add/2
  Reactor Level to High/1(ISD) -> Add/3
  Reactor Level to Low/1(ISD) -> Add/4
  Separator Level to High/1(ISD) -> Add/5
  Separator Level to Low/1(ISD) -> Add/6
  Stripper Level to High/1(ISD) -> Add/7
  Stripper Level to Low/1(ISD) -> Add/8
  Add/1 -> [ISD]

== system COSTEP/Stream Measurements ==
  Stream Variables : ToWorkspace  VariableName=SM  SampleTime=-1
  Subsystem6 : Subsystem
      mask Display: image('$imagefile'); % Use "Edit Image" on toolstrip to change.
  wires:
  Subsystem6/1(SM) -> Stream Variables/1

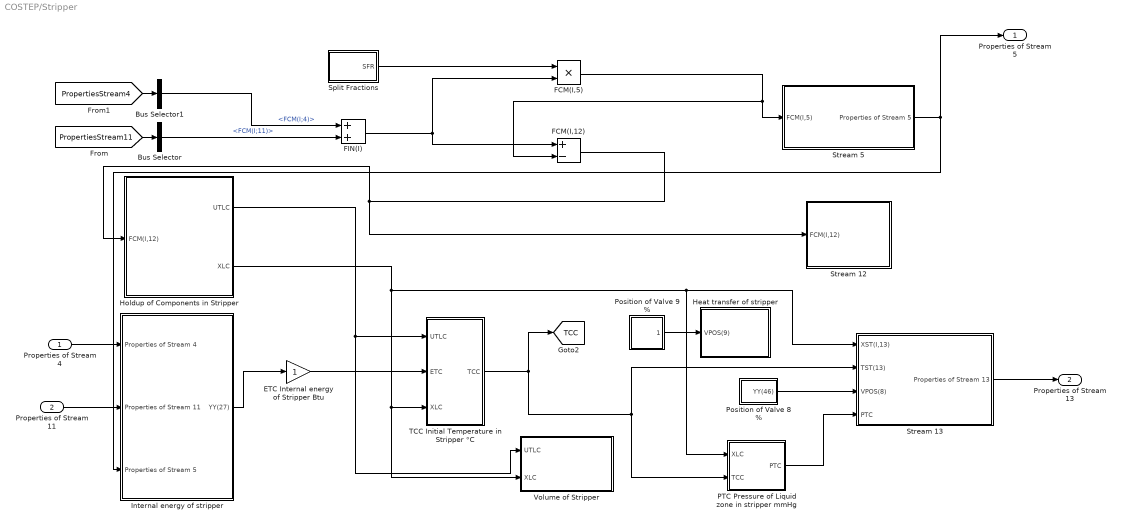
== system COSTEP/Stripper ==
  Properties of Stream 4 : Inport
  Properties of Stream 11 : Inport  Port=2
  Bus Selector : BusSelector  OutputSignals=signal1.FCM(I;11)
  Bus Selector1 : BusSelector  OutputSignals=FCM(I;4)
  ETC Internal energy of Stripper Btu : Gain
  FCM(I,12) : Sum  Inputs=+-
  FCM(I,5) : Product
  FIN(I) : Sum
  Heat transfer of stripper : Subsystem
  Holdup of Components in Stripper : Subsystem
  Internal energy of stripper : Subsystem
  PTC Pressure of Liquid zone in stripper mmHg : Subsystem
  Position of Valve 8 % : Subsystem
  Position of Valve 9 % : Subsystem
  Split Fractions : Subsystem
  Stream 12 : Subsystem
  Stream 13 : Subsystem
  Stream 5 : Subsystem
  "TCC Initial Temperature in Stripper °C " : Subsystem
  Volume of Stripper : Subsystem
  Properties of Stream 5 : Outport  VectorParamsAs1DForOutWhenUnconnected=off
  Properties of Stream 13 : Outport  Port=2  VectorParamsAs1DForOutWhenUnconnected=off
  tag scope: TCC=global
  wires:
  Holdup of Components in Stripper/1(UTLC) -> Volume of Stripper/1(UTLC), "TCC Initial Temperature in Stripper °C "/1(UTLC)
  Internal energy of stripper/1("YY(27) ") -> ETC Internal energy of Stripper Btu/1
  ETC Internal energy of Stripper Btu/1 -> "TCC Initial Temperature in Stripper °C "/2(ETC)
  "TCC Initial Temperature in Stripper °C "/1(TCC) -> [TCC], Stream 13/2(TST(13)), PTC Pressure of Liquid zone in stripper mmHg/2(TCC)
  FIN(I)/1 -> FCM(I,12)/1, FCM(I,5)/2
  FCM(I,5)/1 -> FCM(I,12)/2, Stream 5/1(FCM(I,5))
  FCM(I,12)/1 -> Holdup of Components in Stripper/1("FCM(I,12) "), Stream 12/1(FCM(I,12))
  Stream 13/1(Properties of Stream 13) -> Properties of Stream 13/1
  Stream 5/1(Properties of Stream 5) -> Properties of Stream 5/1, Internal energy of stripper/3(Properties of Stream 5)
  Properties of Stream 4/1 -> Internal energy of stripper/1(Properties of Stream 4)
  Properties of Stream 11/1 -> Internal energy of stripper/2(Properties of Stream 11)
  Position of Valve 9 %/1("YY(47) ") -> Heat transfer of stripper/1(VPOS(9))
  Split Fractions/1(SFR) -> FCM(I,5)/1
  [PropertiesStream11] -> Bus Selector/1
  Bus Selector/1 -> FIN(I)/2  "<FCM(I;11)>"
  [PropertiesStream4] -> Bus Selector1/1
  Bus Selector1/1 -> FIN(I)/1  "<FCM(I;4)>"
  Position of Valve 8 %/1("YY(46) ") -> Stream 13/3(VPOS(8))
  Holdup of Components in Stripper/2(XLC) -> "TCC Initial Temperature in Stripper °C "/3(XLC), Volume of Stripper/2(XLC), PTC Pressure of Liquid zone in stripper mmHg/1(XLC), Stream 13/1(XST(I,13))
  PTC Pressure of Liquid zone in stripper mmHg/1(PTC) -> Stream 13/4(PTC)

== system COSTEP/Valve ==
  Properties of Feed D : Inport
  Bus Creator : BusCreator  Inputs=5
  Bus Selector : BusSelector  OutputSignals=VRNG(1)
  Bus Selector1 : BusSelector  OutputSignals=XST(I;1),TST(1),HST(1)
  FCM(I,1) Component molar flow of Stream 1 lb-mol/h : Product  OutDataTypeStr=Inherit: Same as first input
  FTM(1) Total molar flow of Stream 1 lb-mol/h : Subsystem
  Position of Valve 1 % : Subsystem
  Properties of Stream 1 : Outport  VectorParamsAs1DForOutWhenUnconnected=off
  tag scope: PropertiesStream1=global
  wires:
  Position of Valve 1 %/1("YY(39) ") -> FTM(1) Total molar flow of Stream 1 lb-mol/h/1(VPOS(1))
  Properties of Feed D/1 -> Bus Selector1/1, Bus Selector/1
  Bus Selector/1 -> FTM(1) Total molar flow of Stream 1 lb-mol/h/2(VRNG(1))  "<VRNG(1)>"
  Bus Selector1/1 -> Bus Creator/1, FCM(I,1) Component molar flow of Stream 1 lb-mol/h/1  "<XST(I;1)>"
  FTM(1) Total molar flow of Stream 1 lb-mol/h/1(FTM(1)) -> Bus Creator/4, FCM(I,1) Component molar flow of Stream 1 lb-mol/h/2  "FTM(1)"
  Bus Selector1/2 -> Bus Creator/2  "<TST(1)>"
  Bus Selector1/3 -> Bus Creator/3  "<HST(1)>"
  FCM(I,1) Component molar flow of Stream 1 lb-mol/h/1 -> Bus Creator/5  "FCM(I;1)"
  Bus Creator/1 -> [PropertiesStream1], Properties of Stream 1/1

== system COSTEP/Valve 2 ==
  Properties of Feed E : Inport
  Bus Creator : BusCreator  Inputs=5
  Bus Selector : BusSelector  OutputSignals=VRNG(2)
  Bus Selector1 : BusSelector  OutputSignals=XST(I;2),TST(2),HST(2)
  FCM(I,2) Component molar flow of Stream 2 lb-mol/h : Product
  FTM(2) Total molar flow of Stream 2 lb-mol/h : Subsystem
  Position of Valve 2 % : Subsystem
  Properties of Stream 2 : Outport  VectorParamsAs1DForOutWhenUnconnected=off
  tag scope: PropertiesStream2=global
  wires:
  Properties of Feed E/1 -> Bus Selector1/1, Bus Selector/1
  Bus Selector/1 -> FTM(2) Total molar flow of Stream 2 lb-mol/h/2(VRNG(2))  "<VRNG(2)>"
  Bus Selector1/1 -> Bus Creator/1, FCM(I,2) Component molar flow of Stream 2 lb-mol/h/1  "<XST(I;2)>"
  FTM(2) Total molar flow of Stream 2 lb-mol/h/1(FTM(2)) -> Bus Creator/4, FCM(I,2) Component molar flow of Stream 2 lb-mol/h/2  "FTM(2)"
  Bus Selector1/2 -> Bus Creator/2  "<TST(2)>"
  Bus Selector1/3 -> Bus Creator/3  "<HST(2)>"
  FCM(I,2) Component molar flow of Stream 2 lb-mol/h/1 -> Bus Creator/5  "FCM(I;2)"
  Bus Creator/1 -> [PropertiesStream2], Properties of Stream 2/1
  Position of Valve 2 %/1("YY(40)  ") -> FTM(2) Total molar flow of Stream 2 lb-mol/h/1(VPOS(2))

== system COSTEP/Valve 3 ==
  Properties of Feed A : Inport
  Bus Creator : BusCreator  Inputs=5
  Bus Selector : BusSelector  OutputSignals=VRNG(3)
  Bus Selector1 : BusSelector  OutputSignals=XST(I;3),TST(3),HST(3)
  FCM(I,3) Component molar flow of Stream 3 lb-mol/h : Product
  FTM(3) Total molar flow of Stream 3 lb-mol/h : Subsystem
  Position of Valve 3 % : Subsystem
  Properties of Stream 3 : Outport  VectorParamsAs1DForOutWhenUnconnected=off
  tag scope: PropertiesStream3=global
  wires:
  Properties of Feed A/1 -> Bus Selector1/1, Bus Selector/1
  Bus Selector/1 -> FTM(3) Total molar flow of Stream 3 lb-mol/h/2(VRNG(3))  "<VRNG(3)>"
  Bus Selector1/1 -> Bus Creator/1, FCM(I,3) Component molar flow of Stream 3 lb-mol/h/1  "<XST(I;3)>"
  FTM(3) Total molar flow of Stream 3 lb-mol/h/1(FTM(3)) -> Bus Creator/4, FCM(I,3) Component molar flow of Stream 3 lb-mol/h/2  "FTM(3)"
  Bus Selector1/2 -> Bus Creator/2  "<TST(3)>"
  Bus Selector1/3 -> Bus Creator/3  "<HST(3)>"
  FCM(I,3) Component molar flow of Stream 3 lb-mol/h/1 -> Bus Creator/5  "FCM(I;3)"
  Bus Creator/1 -> [PropertiesStream3], Properties of Stream 3/1
  Position of Valve 3 %/1("YY(41) ") -> FTM(3) Total molar flow of Stream 3 lb-mol/h/1(VPOS(3))

== system COSTEP/Valve 4 ==
  Properties of Feed C : Inport
  Bus Creator : BusCreator  Inputs=5
  Bus Selector : BusSelector  OutputSignals=VRNG(4)
  Bus Selector1 : BusSelector  OutputSignals=XST(I;4),TST(4),HST(4)
  FCM(I,4) Component molar flow of Stream 4 lb-mol/h : Product
  FTM(4) Total molar flow of Stream 4 lb-mol/h : Subsystem
  Position of Valve 4 % : Subsystem
  Properties of Stream 4 : Outport  VectorParamsAs1DForOutWhenUnconnected=off
  tag scope: PropertiesStream4=global
  wires:
  Properties of Feed C/1 -> Bus Selector1/1, Bus Selector/1
  Bus Selector/1 -> FTM(4) Total molar flow of Stream 4 lb-mol/h/2(VRNG(4))  "<VRNG(4)>"
  Bus Selector1/1 -> Bus Creator/1, FCM(I,4) Component molar flow of Stream 4 lb-mol/h/1  "<XST(I;4)>"
  FTM(4) Total molar flow of Stream 4 lb-mol/h/1(FTM(4)) -> Bus Creator/4, FCM(I,4) Component molar flow of Stream 4 lb-mol/h/2  "FTM(4)"
  Bus Selector1/2 -> Bus Creator/2  "<TST(4)>"
  Bus Selector1/3 -> Bus Creator/3  "<HST(4)>"
  FCM(I,4) Component molar flow of Stream 4 lb-mol/h/1 -> Bus Creator/5  "FCM(I;4)"
  Bus Creator/1 -> [PropertiesStream4], Properties of Stream 4/1
  Position of Valve 4 %/1("YY(42) ") -> FTM(4) Total molar flow of Stream 4 lb-mol/h/1(VPOS(4))

== system COSTEP/A Feed Stream/HST(3) Molar Enthalpy of Stream 3 MBtu//lb-mol ==
  TST(3) : Inport
  XST(I,3) : Inport  Port=2
  "Enthalpy of Stream " : mylib/Enthalpy of Stream   SystemSampleTime=-1  VariantActivationTime=update diagram  AllowFlexibleInterface=on  Latency=0  AutoFrameSizeCalculation=off
  ITY : Constant
  HST(3) : Outport  VectorParamsAs1DForOutWhenUnconnected=off
  wires:
  ITY/1 -> "Enthalpy of Stream "/1
  TST(3)/1 -> "Enthalpy of Stream "/2
  XST(I,3)/1 -> "Enthalpy of Stream "/3
  "Enthalpy of Stream "/1 -> HST(3)/1

== system COSTEP/A Feed Stream/TST(3) Temperature of Stream 3 °C ==
  Bus Selector : BusSelector  OutputSignals=signal3.TESUB8(13)
  TST(3) : Outport  PortDimensions=1  VectorParamsAs1DForOutWhenUnconnected=off
  wires:
  [TESUB8] -> Bus Selector/1
  Bus Selector/1 -> TST(3)/1  "<TESUB8(13)>"

== system COSTEP/A Feed Stream/VRNG(3) Max flow of Stream 3 through valve lb-mol//h ==
  Bus Selector : BusSelector  OutputSignals=signal3.TESUB8(15)
  VRNG(3) : Outport  PortDimensions=1  VectorParamsAs1DForOutWhenUnconnected=off
  wires:
  [TESUB8] -> Bus Selector/1
  Bus Selector/1 -> VRNG(3)/1  "<TESUB8(15)>"

== system COSTEP/A//B//C Feed Stream/HST(4) Molar Enthalpy of Stream 4 MBtu//lb-mol ==
  TST(4) : Inport
  XST(I,4) : Inport  Port=2
  "Enthalpy of Stream " : mylib/Enthalpy of Stream   SystemSampleTime=-1  VariantActivationTime=update diagram  AllowFlexibleInterface=on  Latency=0  AutoFrameSizeCalculation=off
  ITY : Constant
  HST(4) : Outport  VectorParamsAs1DForOutWhenUnconnected=off
  wires:
  ITY/1 -> "Enthalpy of Stream "/1
  TST(4)/1 -> "Enthalpy of Stream "/2
  XST(I,4)/1 -> "Enthalpy of Stream "/3
  "Enthalpy of Stream "/1 -> HST(4)/1

== system COSTEP/A//B//C Feed Stream/VRNG(4) Max flow of Stream 4 through valve lb-mol//h ==
  Bus Selector : BusSelector  OutputSignals=signal3.TESUB8(18)
  VRNG(4) : Outport  PortDimensions=1  VectorParamsAs1DForOutWhenUnconnected=off
  wires:
  [TESUB8] -> Bus Selector/1
  Bus Selector/1 -> VRNG(4)/1  "<TESUB8(18)>"

== system COSTEP/A//B//C Feed Stream/XST(I;4) Composition of Stream 4  ==
  TESUB8(1) : Inport
  TESUB8(2) : Inport  Port=2
  IDV(1) : Inport  Port=3
  IDV(2) : Inport  Port=4
  Bus Creator : BusCreator  Inputs=4
  Bus to Vector : BusToVector
  Constant1 : Constant  Value=2.43719e-3
  Constant3 : Constant
  Constant4 : Constant  Value=[XST4_D;XST4_E;XST4_F;XST4_G;XST4_H]
  Gain : Gain  Gain=0.03
  Gain1 : Gain  Gain=0.005
  Product1 : Product
  XST(1,4) : Sum  Inputs=+--
  XST(2,4) : Sum
  XST(3,4) : Sum  Inputs=+--
  XST(I;4) : Outport  PortDimensions=8  VectorParamsAs1DForOutWhenUnconnected=off
  wires:
  TESUB8(1)/1 -> XST(1,4)/1
  XST(1,4)/1 -> Bus Creator/1, XST(3,4)/2
  Product1/1 -> XST(1,4)/3
  IDV(1)/1 -> Gain/1
  Constant3/1 -> XST(3,4)/1
  Gain/1 -> XST(1,4)/2
  XST(2,4)/1 -> Bus Creator/2, XST(3,4)/3
  IDV(2)/1 -> Gain1/1, Product1/1
  Constant1/1 -> Product1/2
  TESUB8(2)/1 -> XST(2,4)/1
  Gain1/1 -> XST(2,4)/2
  XST(3,4)/1 -> Bus Creator/3
  Constant4/1 -> Bus Creator/4
  Bus Creator/1 -> Bus to Vector/1
  Bus to Vector/1 -> XST(I;4)/1

== system COSTEP/Compressor/   ==
  PR : Inport
  CPFLMX : Inport  Port=2
  FLCOEF : Inport  Port=3
  " " : Constant
  "   " : Constant  Value=3
  Add : Sum
  Math Function : Math  Operator=pow  SignedPower=on
  Product : Product
  Subtract : Sum  Inputs=+-
  FLMS : Outport  VectorParamsAs1DForOutWhenUnconnected=off
  wires:
  CPFLMX/1 -> Add/1
  Math Function/1 -> Subtract/2
  PR/1 -> Math Function/1
  " "/1 -> Subtract/1
  Add/1 -> FLMS/1
  FLCOEF/1 -> Product/2
  "   "/1 -> Math Function/2
  Product/1 -> Add/2
  Subtract/1 -> Product/1

== system COSTEP/Compressor/CPDH Compressor work MBtu//h ==
  FLMS : Inport
  TKS : Inport  Port=2
  "XMWS(9) " : Inport  Port=3
  "Convert Btu/°R to MBtu/K " : Constant  Value=1.8e-6
  Divide : Product  Inputs=*/
  PTV-PTS : Sum  Inputs=+-
  Product : Product  Inputs=5
  Product1 : Product
  Universal gas constant Btu/lb-mol·°R : Constant  Value=1.9872
  CPDH : Outport  PortDimensions=1  VectorParamsAs1DForOutWhenUnconnected=off
  wires:
  "Convert Btu/°R to MBtu/K "/1 -> Product/3
  [PTS] -> Product1/2, PTV-PTS/2
  TKS/1 -> Product/2
  Universal gas constant Btu/lb-mol·°R/1 -> Product/4
  Product1/1 -> Divide/2
  Product/1 -> Divide/1
  PTV-PTS/1 -> Product/5
  FLMS/1 -> Product/1
  "XMWS(9) "/1 -> Product1/1
  [PTV] -> PTV-PTS/1
  Divide/1 -> CPDH/1

== system COSTEP/Compressor/Subsystem ==
  CPPRMX : Constant  Value=1.3
  If : If  IfExpression=u1 < 1  ElseIfExpressions=u1>1.3
  If Action Subsystem : Subsystem  TreatAsAtomicUnit=on
  If Action Subsystem1 : Subsystem  TreatAsAtomicUnit=on
  If Action Subsystem2 : Subsystem  TreatAsAtomicUnit=on
  Merge : Merge  Inputs=3
  Minimum Pressure Ratio : Constant
  PR Pressure Ratio : Product  Inputs=*/
  PR : Outport  VectorParamsAs1DForOutWhenUnconnected=off
  wires:
  [PTS] -> PR Pressure Ratio/2
  PR Pressure Ratio/1 -> If Action Subsystem2/1(In1), If/1
  [PTV] -> PR Pressure Ratio/1
  If Action Subsystem1/1(Out1) -> Merge/2
  If Action Subsystem/1(Out1) -> Merge/1
  If/3 -> If Action Subsystem2/Action
  CPPRMX/1 -> If Action Subsystem1/1(In1)
  Minimum Pressure Ratio/1 -> If Action Subsystem/1(In1)
  If/2 -> If Action Subsystem1/Action
  If/1 -> If Action Subsystem/Action
  If Action Subsystem2/1(Out1) -> Merge/3
  Merge/1 -> PR/1

== system COSTEP/Compressor/Subsystem1 ==
  CPFLMX : Inport
  " " : Constant  Value=1.197
  Divide : Product  Inputs=*/
  FLCOEF : Outport  VectorParamsAs1DForOutWhenUnconnected=off
  wires:
  " "/1 -> Divide/2
  Divide/1 -> FLCOEF/1
  CPFLMX/1 -> Divide/1

== system COSTEP/Condenser/Cooling water outlet temperature ==
  FWS : Inport
  QUS : Inport  Port=2
  Constant : Constant  Value=38
  Constant1 : Constant  Value=1e6
  Constant2 : Constant  Value=1.8
  Constant6 : Constant  Value=500.53
  Divide : Product  Inputs=*/
  Divide1 : Product
  Divide2 : Product  Inputs=*/
  HWS : Constant  Value=11138
  Initial state variable : mylib/Initial state variable
  Integration : mylib/Integration  SystemSampleTime=-1  VariantActivationTime=update diagram  AllowFlexibleInterface=on  Latency=0  AutoFrameSizeCalculation=off
  Product : Product  Inputs=3
  Subtract : Sum  Inputs=+-
  TCWS Inlet temperature of cooling water °C : Subsystem
  TCWS-TWS : Sum  Inputs=+-
  "YY(38) " : Outport  VectorParamsAs1DForOutWhenUnconnected=off
  tag scope: TCWS=global, TWS=global
  wires:
  Divide2/1 -> Integration/1
  Initial state variable/1 -> Integration/2
  TCWS Inlet temperature of cooling water °C/1(TCWS) -> [TCWS], TCWS-TWS/1
  Integration/1 -> [TWS], "YY(38) "/1, TCWS-TWS/2
  FWS/1 -> Product/1
  Constant6/1 -> Product/2
  TCWS-TWS/1 -> Product/3
  QUS/1 -> Divide1/1
  Constant1/1 -> Divide1/2
  Divide1/1 -> Divide/1
  Constant2/1 -> Divide/2
  Product/1 -> Subtract/1
  Divide/1 -> Subtract/2
  Subtract/1 -> Divide2/1
  HWS/1 -> Divide2/2
  Constant/1 -> Initial state variable/1

== system COSTEP/Condenser/FWS Flow of cooling water to Condenser Gallons per minute ==
  VPOS(11) : Inport
  VRNG(11) : Inport  Port=2
  " " : Product  Inputs=**/
  Constant2 : Constant  Value=100
  FWS : Outport  VectorParamsAs1DForOutWhenUnconnected=off
  wires:
  Constant2/1 -> " "/3
  " "/1 -> FWS/1
  VPOS(11)/1 -> " "/1
  VRNG(11)/1 -> " "/2

== system COSTEP/Condenser/Position of Valve 11 % ==
  Bus Selector : BusSelector  OutputSignals=XMV(11)
  Bus Selector1 : BusSelector  OutputSignals=IDV(15)
  Constant : Constant  Value=49
  Control valve : mylib/Control valve  SystemSampleTime=-1  VariantActivationTime=update diagram  AllowFlexibleInterface=on  Latency=0  AutoFrameSizeCalculation=off
  Divide : Product  Inputs=*/
  Initial state variable : mylib/Initial state variable
  Integration : mylib/Integration  SystemSampleTime=-1  VariantActivationTime=update diagram  AllowFlexibleInterface=on  Latency=0  AutoFrameSizeCalculation=off
  Subtract : Sum  Inputs=+-
  VTAU(11) : Constant  Value=5/3600
  "YY(49) " : Outport  PortDimensions=1  VectorParamsAs1DForOutWhenUnconnected=off
  wires:
  Integration/1 -> "YY(49) "/1, Subtract/2  "VPOS(11)"
  Subtract/1 -> Divide/1
  Control valve/1 -> Subtract/1
  VTAU(11)/1 -> Divide/2
  Divide/1 -> Integration/1
  Initial state variable/1 -> Integration/2
  [XMV] -> Bus Selector/1
  Bus Selector/1 -> Control valve/1  "<XMV(11)>"
  Bus Selector1/1 -> Control valve/2  "<IDV(15)>"
  [IDV] -> Bus Selector1/1
  Constant/1 -> Initial state variable/1
